simulink model "Solar_cell_model_new"  (R2021a)
settings: Solver=VariableStepAuto  StartTime=0.0  StopTime=10.0  RelTol=1e-3
settings Model: Creator=USER  LastModifiedBy=USER

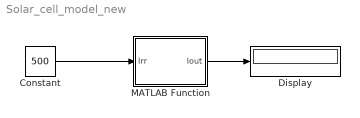
== system Solar_cell_model_new ==
  Constant : Constant  Value=500
  Display : Display
  MATLAB Function : MATLAB Function  TreatAsAtomicUnit=on
  wires:
  MATLAB Function/1(Iout) -> Display/1
  Constant/1 -> MATLAB Function/1(Irr)

== matlab function Solar_cell_model_new/MATLAB Function ==
  data: Irr input; Iout output
function Iout = solar_fcn(Irr)
e = 1.6e-19; 
kb = 1.38e-23;

T = 300; % temperature in kelvin
I0 = 25e-9; %reverse saturation current(A)
%Iph = 10e-3; %Photocurrent of the solar cell(A)
K = 2e-5; % for Si solar cell
Iph = K*Irr; 
Eg = 1.14; % Bandgap of Si
n = 1; %Ideality factor
Rs = 10; %series resistance of the equivalent model
Rp = 1e6; %parallel resistance of the equivalent model

T_new = 290;
I0_old = I0;
I0=((T_new^3)*exp(Eg./(kb*T_new/e)))*I0/((T^3)*exp(Eg/(kb*T/e))); %reverse saturation current(A)

V=0:0.001:0.4;
I_total = zeros(1,length(V));
for i = 1:length(V)
    fcn = @(I) -I - Iph + I0*(exp(e*(V(i)-I*Rs)/(n*kb*T))-1) + (V(i)-I*Rs)/Rp;
    I = fzero(fcn,Iph);
    I_total(i)= I;
end
Power = (-I_total.*V);

R = 30;
err = (-V/R-I_total);
index = find(abs(err)<0.05e-3);
Iout  = I_total(index)*1e3; % in mA

end
